simulink model "RaibertControlV9"  (R2022a)
settings: Solver=ode23t  StartTime=0.0  StopTime=10  FixedStep=1/1000  MaxStep=0.001  RelTol=1e-3  AbsTol=1e-3  EnableMultiTasking=on
values from neighbouring files (symbols this model uses):
  dphi_d_14 = 0.0    (= 0)    [initialization.m]
  dphi_d_23 = 0.0    (= 0)    [initialization.m]
  dphi_des = DesiredImpedenceValues(4)    [Controller.m]    (also in initialization.m = 0)
  dr_d_14 = 0.0    (= 0)    [initialization.m]
  dr_d_23 = 0.0    (= 0)    [initialization.m]
  dr_des = DesiredImpedenceValues(3)    [Controller.m]    (also in initialization.m = 0)
  Fpush_d_14 = 300    [initialization.m]
  Fpush_d_23 = 300    [initialization.m]
  GAIN_dx_d_14 = 0.05    [initialization.m]
  GAIN_dx_d_23 = 0.05    [initialization.m]
  Kd_phi_d_14 = 10    [initialization.m]
  Kd_phi_d_23 = 10    [initialization.m]
  Kd_r_d_14 = Kp_r_d_14*0.1    (= 60)    [initialization.m]
  Kd_r_d_23 = Kp_r_d_23*0.1    (= 50)    [initialization.m]
  Kdphi_des = DesiredImpedenceValues(8)    [Controller.m]    (also in initialization.m = 5)
  Kdr_des = DesiredImpedenceValues(6)    [Controller.m]    (also in initialization.m = 700)
  Kp_phi_d_14 = 200    [initialization.m]
  Kp_phi_d_23 = 200    [initialization.m]
  Kp_r_d_14 = 600    [initialization.m]
  Kp_r_d_23 = 500    [initialization.m]
  Kpphi_des = DesiredImpedenceValues(7)    [Controller.m]    (also in initialization.m = 50)
  Kpr_des = DesiredImpedenceValues(5)    [Controller.m]    (also in initialization.m = 700)
  phi_d_14 = 0    [initialization.m]
  phi_d_23 = 0    [initialization.m]
  phi_des = DesiredImpedenceValues(2)    [Controller.m]    (also in initialization.m = 0)
  r_d_14 = 0.38    [initialization.m]
  r_d_23 = 0.38    [initialization.m]
  r_des = DesiredImpedenceValues(1)    [Controller.m]    (also in initialization.m = 0.4)
  rthrust_d_14 = 0.3    [initialization.m]
  rthrust_d_23 = 0.3    [initialization.m]
undefined symbols (not defined in the file or in its folder): Carrier, N, Ring, T, X, Y, Z
libraries: sm_lib x133, nesl_utility x26, Multibody_Parts_Lib x4, fl_lib x4
(part 2 of 8)

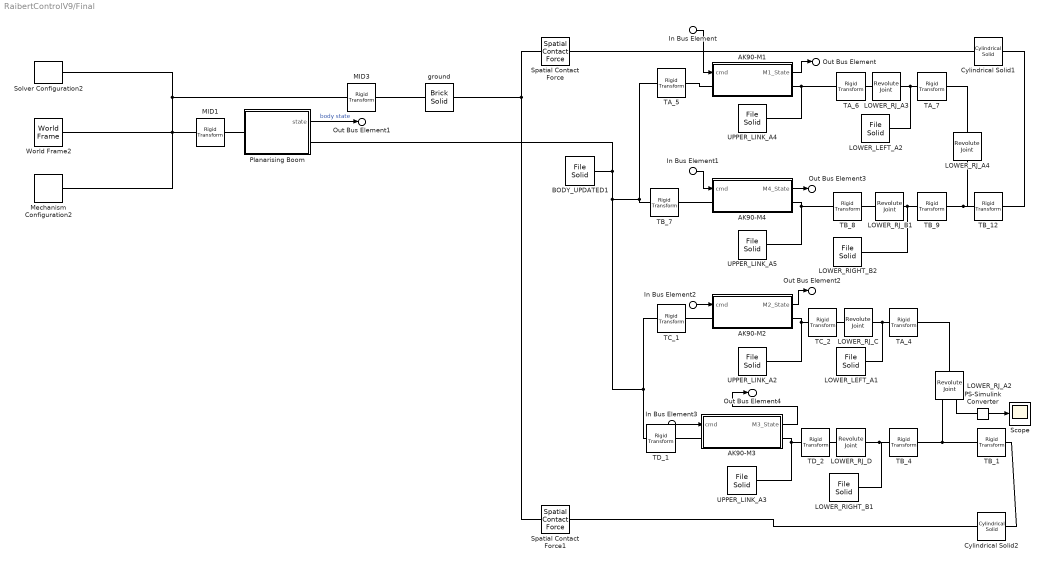
== system RaibertControlV9/Final ==
  In Bus Element1 : Inport  PortName=cmd_M4
  In Bus Element : Inport  Port=2  PortName=cmd_M1
  In Bus Element3 : Inport  Port=3  PortName=cmd_M3
  In Bus Element2 : Inport  Port=4  PortName=cmd_M2
  AK90-M1 : Subsystem
  AK90-M2 : Subsystem
  AK90-M3 : Subsystem
  AK90-M4 : Subsystem
  BODY_UPDATED1 : sm_lib/Body Elements/File Solid  ExtGeomFileName=C:\Users\user\Desktop\Zubair\solidworks_simscape_setup\Rigid Bodies\updated\simscape files\Body.STL  UnitType=Custom  ExtGeomFileUnits=mm  StepReaderType=HEX  ExportConvexHullGeometry=off  InertiaType=Custom  Mass=5756.78  MassUnits=g  CenterOfMass=[0.00 8.34 76.00]  CenterOfMassUnits=mm  MomentsOfInertia="[19417888.32  38930926.54 32124078.52]"  MomentsOfInertiaUnits=g*mm^2  ProductsOfInertia=[0.00 522.32 0.00]  ProductsOfInertiaUnits=g*mm^2  BasedOnType=DensityFromFile  Density=1000  DensityUnits=kg/m^3  DoExposeReferenceFrame=on  SerializedFrames=<Frames/>  GraphicType=FromGeometry  MarkerShape=Sphere  MarkerSize=10  GraphicVisPropType=SimpleVisualProperties  GraphicDiffuseColor=[1.0 1.0 1.0]  GraphicSpecularColor=[0.5 0.5 0.5 1.0]  GraphicAmbientColor=[0.15 0.15 0.15 1.0]  GraphicEmissiveColor=[0.0 0.0 0.0 1.0]  GraphicShininess=75  GraphicOpacity=0.5
  Cylindrical Solid1 : sm_lib/Body Elements/Cylindrical Solid  GraphicAmbientColor=[0.15 0.15 0.15 1.0]  BasedOnType=Density  CenterOfMass=[0 0 0]  CenterOfMassUnits=m  GraphicDiffuseColor=[0.5 0.5 0.5]  CylinderLength=16.25*2  CylinderLengthUnits=mm  CylinderRadius=16.25  CylinderRadiusUnits=mm  Density=1000  DensityUnits=kg/m^3  DoExposeReferenceFrame=on  GraphicEmissiveColor=[0.0 0.0 0.0 1.0]  ExportEntireGeometry=on  SerializedFrames=<Frames/>  MarkerShape=Sphere  MarkerSize=10  GraphicType=FromGeometry  InertiaType=Custom  Mass=0  MassUnits=kg  MomentsOfInertia=[1 1 1]  MomentsOfInertiaUnits=kg*m^2  GraphicOpacity=1.0  ProductsOfInertia=[0 0 0]  ProductsOfInertiaUnits=kg*m^2  GraphicShininess=75  GraphicSpecularColor=[0.5 0.5 0.5 1.0]  GraphicVisPropType=SimpleVisualProperties
  Cylindrical Solid2 : sm_lib/Body Elements/Cylindrical Solid  GraphicAmbientColor=[0.15 0.15 0.15 1.0]  BasedOnType=Density  CenterOfMass=[0 0 0]  CenterOfMassUnits=m  GraphicDiffuseColor=[0.5 0.5 0.5]  CylinderLength=16.25*2  CylinderLengthUnits=mm  CylinderRadius=16.25  CylinderRadiusUnits=mm  Density=1000  DensityUnits=kg/m^3  DoExposeReferenceFrame=on  GraphicEmissiveColor=[0.0 0.0 0.0 1.0]  ExportEntireGeometry=on  SerializedFrames=<Frames/>  MarkerShape=Sphere  MarkerSize=10  GraphicType=FromGeometry  InertiaType=Custom  Mass=0  MassUnits=kg  MomentsOfInertia=[1 1 1]  MomentsOfInertiaUnits=kg*m^2  GraphicOpacity=1.0  ProductsOfInertia=[0 0 0]  ProductsOfInertiaUnits=kg*m^2  GraphicShininess=75  GraphicSpecularColor=[0.5 0.5 0.5 1.0]  GraphicVisPropType=SimpleVisualProperties
  LOWER_LEFT_A1 : sm_lib/Body Elements/File Solid  ExtGeomFileName=C:\Users\user\Desktop\Zubair\solidworks_simscape_setup\Rigid Bodies\updated\simscape files\leg2.STL  UnitType=Custom  ExtGeomFileUnits=mm  StepReaderType=HEX  ExportConvexHullGeometry=off  InertiaType=Custom  Mass=346.45  MassUnits=g  CenterOfMass=[0.00 -132.20 0.00]  CenterOfMassUnits=mm  MomentsOfInertia=[4857689.47 249818.51 4659658.63]  MomentsOfInertiaUnits=g*mm^2  ProductsOfInertia=[0.00 -0.09 10.78]  ProductsOfInertiaUnits=g*mm^2  BasedOnType=DensityFromFile  Density=1000  DensityUnits=kg/m^3  DoExposeReferenceFrame=on  SerializedFrames=<Frames/>  GraphicType=FromGeometry  MarkerShape=Sphere  MarkerSize=10  GraphicVisPropType=SimpleVisualProperties  GraphicDiffuseColor=[1.0 1.0 1.0]  GraphicSpecularColor=[0.5 0.5 0.5 1.0]  GraphicAmbientColor=[0.15 0.15 0.15 1.0]  GraphicEmissiveColor=[0.0 0.0 0.0 1.0]  GraphicShininess=75  GraphicOpacity=1.0
  LOWER_LEFT_A2 : sm_lib/Body Elements/File Solid  ExtGeomFileName=C:\Users\user\Desktop\Zubair\solidworks_simscape_setup\Rigid Bodies\updated\simscape files\leg2.STL  UnitType=Custom  ExtGeomFileUnits=mm  StepReaderType=HEX  ExportConvexHullGeometry=off  InertiaType=Custom  Mass=346.45  MassUnits=g  CenterOfMass=[0.00 -132.20 0.00]  CenterOfMassUnits=mm  MomentsOfInertia=[4857689.47 249818.51 4659658.63]  MomentsOfInertiaUnits=g*mm^2  ProductsOfInertia=[0.00 -0.09 10.78]  ProductsOfInertiaUnits=g*mm^2  BasedOnType=DensityFromFile  Density=1000  DensityUnits=kg/m^3  DoExposeReferenceFrame=on  SerializedFrames=<Frames/>  GraphicType=FromGeometry  MarkerShape=Sphere  MarkerSize=10  GraphicVisPropType=SimpleVisualProperties  GraphicDiffuseColor=[1.0 1.0 1.0]  GraphicSpecularColor=[0.5 0.5 0.5 1.0]  GraphicAmbientColor=[0.15 0.15 0.15 1.0]  GraphicEmissiveColor=[0.0 0.0 0.0 1.0]  GraphicShininess=75  GraphicOpacity=1.0
  LOWER_RIGHT_B1 : sm_lib/Body Elements/File Solid  ExtGeomFileName=C:\Users\user\Desktop\Zubair\solidworks_simscape_setup\Rigid Bodies\updated\simscape files\leg3.STL  UnitType=Custom  ExtGeomFileUnits=mm  StepReaderType=HEX  ExportConvexHullGeometry=off  InertiaType=Custom  Mass=499.95  MassUnits=g  CenterOfMass=[1.63 -190.40 0.00]  CenterOfMassUnits=mm  MomentsOfInertia=[7423471.12 197304.86 7369968.50]  MomentsOfInertiaUnits=g*mm^2  ProductsOfInertia=[2.77 -22.94 255458.86]  ProductsOfInertiaUnits=g*mm^2  BasedOnType=Mass  Density=1000  DensityUnits=kg/m^3  DoExposeReferenceFrame=on  SerializedFrames=<Frames/>  GraphicType=FromGeometry  MarkerShape=Sphere  MarkerSize=10  GraphicVisPropType=SimpleVisualProperties  GraphicDiffuseColor=[1.0 1.0 1.0]  GraphicSpecularColor=[0.5 0.5 0.5 1.0]  GraphicAmbientColor=[0.15 0.15 0.15 1.0]  GraphicEmissiveColor=[0.0 0.0 0.0 1.0]  GraphicShininess=75  GraphicOpacity=1.0
  LOWER_RIGHT_B2 : sm_lib/Body Elements/File Solid  ExtGeomFileName=C:\Users\user\Desktop\Zubair\solidworks_simscape_setup\Rigid Bodies\updated\simscape files\leg3.STL  UnitType=Custom  ExtGeomFileUnits=mm  StepReaderType=HEX  ExportConvexHullGeometry=off  InertiaType=Custom  Mass=499.95  MassUnits=g  CenterOfMass=[1.63 -190.40 0.00]  CenterOfMassUnits=mm  MomentsOfInertia=[7423471.12 197304.86 7369968.50]  MomentsOfInertiaUnits=g*mm^2  ProductsOfInertia=[2.77 -22.94 255458.86]  ProductsOfInertiaUnits=g*mm^2  BasedOnType=Mass  Density=1000  DensityUnits=kg/m^3  DoExposeReferenceFrame=on  SerializedFrames=<Frames/>  GraphicType=FromGeometry  MarkerShape=Sphere  MarkerSize=10  GraphicVisPropType=SimpleVisualProperties  GraphicDiffuseColor=[1.0 1.0 1.0]  GraphicSpecularColor=[0.5 0.5 0.5 1.0]  GraphicAmbientColor=[0.15 0.15 0.15 1.0]  GraphicEmissiveColor=[0.0 0.0 0.0 1.0]  GraphicShininess=75  GraphicOpacity=1.0
  LOWER_RJ_A2 : sm_lib/Joints/Revolute Joint  JointMode=Normal  SenseConstraintForce=off  SenseConstraintForceX=off  SenseConstraintForceY=off  SenseConstraintForceZ=off  SenseConstraintTorque=off  SenseConstraintTorqueX=off  SenseConstraintTorqueY=off  SenseConstraintTorqueZ=off  SenseTotalForce=off  SenseTotalForceX=off  SenseTotalForceY=off  SenseTotalForceZ=off  SenseTotalTorque=off  SenseTotalTorqueX=off  SenseTotalTorqueY=off  SenseTotalTorqueZ=off  CompositeWrenchDir=FollowerOnBase  CompositeWrenchFrame=BaseFrame  EquilibriumPosition=0  EquilibriumPositionUnits=deg  SpringStiffness=0  SpringStiffnessUnits=N*m/deg  DampingCoefficient=0  DampingCoefficientUnits=N*m/(deg/s)  TorqueActuationMode=NoTorque  MotionActuationMode=ComputedMotion  SensePosition=on  SenseVelocity=off  SenseAcceleration=off  SenseTorqueForce=off  SenseLowerLimitTorqueForce=off  SenseUpperLimitTorqueForce=off  LowerLimitSpecify=on  LowerLimitBound=0  LowerLimitBoundUnits=deg  LowerLimitStiffness=1e4  LowerLimitStiffnessUnits=N*m/deg  LowerLimitDamping=10  LowerLimitDampingUnits=N*m/(deg/s)  LowerLimitTransitionRegionWidth=0.1  LowerLimitTransitionRegionWidthUnits=deg  UpperLimitSpecify=off  UpperLimitBound=90  UpperLimitBoundUnits=deg  UpperLimitStiffness=1e4  UpperLimitStiffnessUnits=N*m/deg  UpperLimitDamping=10  UpperLimitDampingUnits=N*m/(deg/s)  UpperLimitTransitionRegionWidth=0.1  UpperLimitTransitionRegionWidthUnits=deg  PositionTargetSpecify=off  PositionTargetPriority=High  PositionTargetValue=10  PositionTargetValueUnits=deg  VelocityTargetSpecify=off  VelocityTargetPriority=High  VelocityTargetValue=0  VelocityTargetValueUnits=deg/s
  LOWER_RJ_A3 : sm_lib/Joints/Revolute Joint  JointMode=Normal  SenseConstraintForce=off  SenseConstraintForceX=off  SenseConstraintForceY=off  SenseConstraintForceZ=off  SenseConstraintTorque=off  SenseConstraintTorqueX=off  SenseConstraintTorqueY=off  SenseConstraintTorqueZ=off  SenseTotalForce=off  SenseTotalForceX=off  SenseTotalForceY=off  SenseTotalForceZ=off  SenseTotalTorque=off  SenseTotalTorqueX=off  SenseTotalTorqueY=off  SenseTotalTorqueZ=off  CompositeWrenchDir=FollowerOnBase  CompositeWrenchFrame=BaseFrame  EquilibriumPosition=0  EquilibriumPositionUnits=deg  SpringStiffness=0  SpringStiffnessUnits=N*m/deg  DampingCoefficient=0  DampingCoefficientUnits=N*m/(deg/s)  TorqueActuationMode=NoTorque  MotionActuationMode=ComputedMotion  SensePosition=off  SenseVelocity=off  SenseAcceleration=off  SenseTorqueForce=off  SenseLowerLimitTorqueForce=off  SenseUpperLimitTorqueForce=off  LowerLimitSpecify=off  LowerLimitBound=-90  LowerLimitBoundUnits=deg  LowerLimitStiffness=1e4  LowerLimitStiffnessUnits=N*m/deg  LowerLimitDamping=10  LowerLimitDampingUnits=N*m/(deg/s)  LowerLimitTransitionRegionWidth=0.1  LowerLimitTransitionRegionWidthUnits=deg  UpperLimitSpecify=off  UpperLimitBound=90  UpperLimitBoundUnits=deg  UpperLimitStiffness=1e4  UpperLimitStiffnessUnits=N*m/deg  UpperLimitDamping=10  UpperLimitDampingUnits=N*m/(deg/s)  UpperLimitTransitionRegionWidth=0.1  UpperLimitTransitionRegionWidthUnits=deg  PositionTargetSpecify=off  PositionTargetPriority=High  PositionTargetValue=10  PositionTargetValueUnits=deg  VelocityTargetSpecify=off  VelocityTargetPriority=High  VelocityTargetValue=0  VelocityTargetValueUnits=deg/s
  LOWER_RJ_A4 : sm_lib/Joints/Revolute Joint  JointMode=Normal  SenseConstraintForce=off  SenseConstraintForceX=off  SenseConstraintForceY=off  SenseConstraintForceZ=off  SenseConstraintTorque=off  SenseConstraintTorqueX=off  SenseConstraintTorqueY=off  SenseConstraintTorqueZ=off  SenseTotalForce=off  SenseTotalForceX=off  SenseTotalForceY=off  SenseTotalForceZ=off  SenseTotalTorque=off  SenseTotalTorqueX=off  SenseTotalTorqueY=off  SenseTotalTorqueZ=off  CompositeWrenchDir=FollowerOnBase  CompositeWrenchFrame=BaseFrame  EquilibriumPosition=0  EquilibriumPositionUnits=deg  SpringStiffness=0  SpringStiffnessUnits=N*m/deg  DampingCoefficient=0  DampingCoefficientUnits=N*m/(deg/s)  TorqueActuationMode=NoTorque  MotionActuationMode=ComputedMotion  SensePosition=off  SenseVelocity=off  SenseAcceleration=off  SenseTorqueForce=off  SenseLowerLimitTorqueForce=off  SenseUpperLimitTorqueForce=off  LowerLimitSpecify=off  LowerLimitBound=0  LowerLimitBoundUnits=deg  LowerLimitStiffness=1e4  LowerLimitStiffnessUnits=N*m/deg  LowerLimitDamping=10  LowerLimitDampingUnits=N*m/(deg/s)  LowerLimitTransitionRegionWidth=0.1  LowerLimitTransitionRegionWidthUnits=deg  UpperLimitSpecify=on  UpperLimitBound=0  UpperLimitBoundUnits=deg  UpperLimitStiffness=1e4  UpperLimitStiffnessUnits=N*m/deg  UpperLimitDamping=10  UpperLimitDampingUnits=N*m/(deg/s)  UpperLimitTransitionRegionWidth=0.1  UpperLimitTransitionRegionWidthUnits=deg  PositionTargetSpecify=off  PositionTargetPriority=High  PositionTargetValue=10  PositionTargetValueUnits=deg  VelocityTargetSpecify=off  VelocityTargetPriority=High  VelocityTargetValue=0  VelocityTargetValueUnits=deg/s
  LOWER_RJ_B1 : sm_lib/Joints/Revolute Joint  JointMode=Normal  SenseConstraintForce=off  SenseConstraintForceX=off  SenseConstraintForceY=off  SenseConstraintForceZ=off  SenseConstraintTorque=off  SenseConstraintTorqueX=off  SenseConstraintTorqueY=off  SenseConstraintTorqueZ=off  SenseTotalForce=off  SenseTotalForceX=off  SenseTotalForceY=off  SenseTotalForceZ=off  SenseTotalTorque=off  SenseTotalTorqueX=off  SenseTotalTorqueY=off  SenseTotalTorqueZ=off  CompositeWrenchDir=FollowerOnBase  CompositeWrenchFrame=BaseFrame  EquilibriumPosition=0  EquilibriumPositionUnits=deg  SpringStiffness=0  SpringStiffnessUnits=N*m/deg  DampingCoefficient=0  DampingCoefficientUnits=N*m/(deg/s)  TorqueActuationMode=NoTorque  MotionActuationMode=ComputedMotion  SensePosition=off  SenseVelocity=off  SenseAcceleration=off  SenseTorqueForce=off  SenseLowerLimitTorqueForce=off  SenseUpperLimitTorqueForce=off  LowerLimitSpecify=off  LowerLimitBound=-90  LowerLimitBoundUnits=deg  LowerLimitStiffness=1e4  LowerLimitStiffnessUnits=N*m/deg  LowerLimitDamping=10  LowerLimitDampingUnits=N*m/(deg/s)  LowerLimitTransitionRegionWidth=0.1  LowerLimitTransitionRegionWidthUnits=deg  UpperLimitSpecify=off  UpperLimitBound=90  UpperLimitBoundUnits=deg  UpperLimitStiffness=1e4  UpperLimitStiffnessUnits=N*m/deg  UpperLimitDamping=10  UpperLimitDampingUnits=N*m/(deg/s)  UpperLimitTransitionRegionWidth=0.1  UpperLimitTransitionRegionWidthUnits=deg  PositionTargetSpecify=off  PositionTargetPriority=High  PositionTargetValue=0  PositionTargetValueUnits=deg  VelocityTargetSpecify=off  VelocityTargetPriority=High  VelocityTargetValue=0  VelocityTargetValueUnits=deg/s
  LOWER_RJ_C : sm_lib/Joints/Revolute Joint  JointMode=Normal  SenseConstraintForce=off  SenseConstraintForceX=off  SenseConstraintForceY=off  SenseConstraintForceZ=off  SenseConstraintTorque=off  SenseConstraintTorqueX=off  SenseConstraintTorqueY=off  SenseConstraintTorqueZ=off  SenseTotalForce=off  SenseTotalForceX=off  SenseTotalForceY=off  SenseTotalForceZ=off  SenseTotalTorque=off  SenseTotalTorqueX=off  SenseTotalTorqueY=off  SenseTotalTorqueZ=off  CompositeWrenchDir=FollowerOnBase  CompositeWrenchFrame=BaseFrame  EquilibriumPosition=0  EquilibriumPositionUnits=deg  SpringStiffness=0  SpringStiffnessUnits=N*m/deg  DampingCoefficient=0  DampingCoefficientUnits=N*m/(deg/s)  TorqueActuationMode=NoTorque  MotionActuationMode=ComputedMotion  SensePosition=off  SenseVelocity=off  SenseAcceleration=off  SenseTorqueForce=off  SenseLowerLimitTorqueForce=off  SenseUpperLimitTorqueForce=off  LowerLimitSpecify=off  LowerLimitBound=-90  LowerLimitBoundUnits=deg  LowerLimitStiffness=1e4  LowerLimitStiffnessUnits=N*m/deg  LowerLimitDamping=10  LowerLimitDampingUnits=N*m/(deg/s)  LowerLimitTransitionRegionWidth=0.1  LowerLimitTransitionRegionWidthUnits=deg  UpperLimitSpecify=off  UpperLimitBound=90  UpperLimitBoundUnits=deg  UpperLimitStiffness=1e4  UpperLimitStiffnessUnits=N*m/deg  UpperLimitDamping=10  UpperLimitDampingUnits=N*m/(deg/s)  UpperLimitTransitionRegionWidth=0.1  UpperLimitTransitionRegionWidthUnits=deg  PositionTargetSpecify=off  PositionTargetPriority=High  PositionTargetValue=10  PositionTargetValueUnits=deg  VelocityTargetSpecify=off  VelocityTargetPriority=High  VelocityTargetValue=0  VelocityTargetValueUnits=deg/s
  LOWER_RJ_D : sm_lib/Joints/Revolute Joint  JointMode=Normal  SenseConstraintForce=off  SenseConstraintForceX=off  SenseConstraintForceY=off  SenseConstraintForceZ=off  SenseConstraintTorque=off  SenseConstraintTorqueX=off  SenseConstraintTorqueY=off  SenseConstraintTorqueZ=off  SenseTotalForce=off  SenseTotalForceX=off  SenseTotalForceY=off  SenseTotalForceZ=off  SenseTotalTorque=off  SenseTotalTorqueX=off  SenseTotalTorqueY=off  SenseTotalTorqueZ=off  CompositeWrenchDir=FollowerOnBase  CompositeWrenchFrame=BaseFrame  EquilibriumPosition=0  EquilibriumPositionUnits=deg  SpringStiffness=0  SpringStiffnessUnits=N*m/deg  DampingCoefficient=0  DampingCoefficientUnits=N*m/(deg/s)  TorqueActuationMode=NoTorque  MotionActuationMode=ComputedMotion  SensePosition=off  SenseVelocity=off  SenseAcceleration=off  SenseTorqueForce=off  SenseLowerLimitTorqueForce=off  SenseUpperLimitTorqueForce=off  LowerLimitSpecify=off  LowerLimitBound=-90  LowerLimitBoundUnits=deg  LowerLimitStiffness=1e4  LowerLimitStiffnessUnits=N*m/deg  LowerLimitDamping=10  LowerLimitDampingUnits=N*m/(deg/s)  LowerLimitTransitionRegionWidth=0.1  LowerLimitTransitionRegionWidthUnits=deg  UpperLimitSpecify=off  UpperLimitBound=90  UpperLimitBoundUnits=deg  UpperLimitStiffness=1e4  UpperLimitStiffnessUnits=N*m/deg  UpperLimitDamping=10  UpperLimitDampingUnits=N*m/(deg/s)  UpperLimitTransitionRegionWidth=0.1  UpperLimitTransitionRegionWidthUnits=deg  PositionTargetSpecify=off  PositionTargetPriority=High  PositionTargetValue=0  PositionTargetValueUnits=deg  VelocityTargetSpecify=off  VelocityTargetPriority=High  VelocityTargetValue=0  VelocityTargetValueUnits=deg/s
  MID1 : sm_lib/Frames and Transforms/Rigid Transform  TranslationMethod=None  TranslationStandardOffset=700  TranslationLengthUnit=mm  TranslationStandardAxis=-Y  TranslationCartesianOffset=[0 0 0]  TranslationROffset=0  TranslationROffsetUnits=m  TranslationZOffset=0  TranslationZOffsetUnits=m  TranslationThetaOffset=0  TranslationThetaOffsetUnits=deg  RotationMethod=StandardAxis  RotationAngleUnits=deg  RotationStandardAxis=+X  RotationAngle=90  RotationArbitraryAxis=[0 0 1]  FollAlignAxisA=+X  BaseAlignAxisA=+Y  FollAlignAxisB=+Y  BaseAlignAxisB=+Z  RotationSequenceAxes=FollowerAxes  RotationSequence=XYX  RotationSequenceAngles=[0 0 0]  RotationSequenceAnglesUnits=deg  RotationMatrix=[1 0 0; 0 1 0; 0 0 1]
  MID3 : sm_lib/Frames and Transforms/Rigid Transform  TranslationMethod=StandardAxis  TranslationStandardOffset=1  TranslationLengthUnit=m  TranslationStandardAxis=-X  TranslationCartesianOffset=[0 0 0]  TranslationROffset=0  TranslationROffsetUnits=m  TranslationZOffset=0  TranslationZOffsetUnits=m  TranslationThetaOffset=0  TranslationThetaOffsetUnits=deg  RotationMethod=StandardAxis  RotationAngleUnits=deg  RotationStandardAxis=+X  RotationAngle=-90  RotationArbitraryAxis=[0 0 1]  FollAlignAxisA=+X  BaseAlignAxisA=+Y  FollAlignAxisB=+Y  BaseAlignAxisB=+Z  RotationSequenceAxes=FollowerAxes  RotationSequence=XYX  RotationSequenceAngles=[0 0 0]  RotationSequenceAnglesUnits=deg  RotationMatrix=[1 0 0; 0 1 0; 0 0 1]
  Mechanism Configuration2 : sm_lib/Utilities/Mechanism Configuration  UniformGravity=Constant  GravityVector=[0 -9.80665 0]  GravityUnits=m/s^2  LinearizationDelta=0.001  JointModeTransitionNonlinearIterations=2
  PS-Simulink Converter : nesl_utility/PS-Simulink Converter  PhysicalDomain=network_engine_domain  SubClassName=ps_output  LeftPortType=input  RightPortType=output  PseudoPeriodic=off  Frequencies=[]  VectorFormat=inherit  Unit=inherit  AffineConversion=off
      settings: SourceProductBaseCode=SS,PW,VE
  Planarising Boom : Subsystem
  Scope : Scope
  Solver Configuration2 : nesl_utility/Solver Configuration  PhysicalDomain=network_engine_domain  SubClassName=solver  LeftPortType=input  RightPortType=generic  Tones=[]  Harmonics=[]  SimulateNoise=off  Profile=off  UseLocalSampling=off  EnableSwitchedLinearOptims=on  FrequencyDomain=off  UseCCode=off  RelTol=0.001  AbsTol=1e-06  MinStep=1e-09  ToWorkspace=off  RevertToSquareIcSolve=off  NumHomotopyIterations=100  PhasorMode=off  PhasorModeNumHarmonics=1  IndexReductionMethod=DerivativeReplacement  DoDC=off  ResidualTolerance=1e-09  UseLocalSolver=off  LocalSolverChoice=NE_BACKWARD_EULER_ADVANCER  LocalSolverSampleTime=0.001  DoFixedCost=off  MaxNonlinIter=3  MaxModeIter=2  ComputeImpulses=off  ImpulseIterations=2  LinearAlgebra=Sparse  LinearAlgebraNumThread=0  EquationFormulation=NE_TIME_EF  DelaysMemoryBudget=1024  AutomaticFiltering=on  FilteringTimeConstant=0.001  PartitionStorageMethod=AS_NEEDED  PartitionMemoryBudget=1024  PartitionMethod=FAST
      settings: SourceProductBaseCode=SS,PW,VE
  Spatial Contact Force : sm_lib/Forces and Torques/Spatial Contact Force  SenseContactBaseRotation=off  SenseContactBaseTranslation=off  CoefficientOfDynamicFriction=0.7  CoefficientOfStaticFriction=0.9  NormalDamping=1e3  NormalDampingUnits=N/(m/s)  SenseContactSignal=off  NormalStiffness=5e4  NormalStiffnessUnits=N/m  FrictionalCriticalVelocity=1e-3  FrictionalCriticalVelocityUnits=m/s  ZeroCrossDetectContactStartAndEnd=on  SenseContactFollowerRotation=off  SenseContactFollowerTranslation=off  FrictionType=SmoothStickSlip  SenseFrictionalForceMagnitude=off  SenseNormalForceMagnitude=off  NormalForceType=SmoothSpringDamper  SenseNormalVelocity=off  SenseSeparationDistance=off  SenseTangentialVelocity=off  NormalTransitionRegionWidth=1e-4  NormalTransitionRegionWidthUnits=m
  Spatial Contact Force1 : sm_lib/Forces and Torques/Spatial Contact Force  SenseContactBaseRotation=off  SenseContactBaseTranslation=off  CoefficientOfDynamicFriction=0.7  CoefficientOfStaticFriction=0.9  NormalDamping=1e3  NormalDampingUnits=N/(m/s)  SenseContactSignal=off  NormalStiffness=5e4  NormalStiffnessUnits=N/m  FrictionalCriticalVelocity=1e-3  FrictionalCriticalVelocityUnits=m/s  ZeroCrossDetectContactStartAndEnd=on  SenseContactFollowerRotation=off  SenseContactFollowerTranslation=off  FrictionType=SmoothStickSlip  SenseFrictionalForceMagnitude=off  SenseNormalForceMagnitude=off  NormalForceType=SmoothSpringDamper  SenseNormalVelocity=off  SenseSeparationDistance=off  SenseTangentialVelocity=off  NormalTransitionRegionWidth=1e-4  NormalTransitionRegionWidthUnits=m
  TA_4 : sm_lib/Frames and Transforms/Rigid Transform  TranslationMethod=Cartesian  TranslationStandardOffset=60  TranslationLengthUnit=mm  TranslationStandardAxis=-X  TranslationCartesianOffset=[0 -300 0]  TranslationROffset=0  TranslationROffsetUnits=m  TranslationZOffset=0  TranslationZOffsetUnits=m  TranslationThetaOffset=0  TranslationThetaOffsetUnits=deg  RotationMethod=None  RotationAngleUnits=deg  RotationStandardAxis=+Z  RotationAngle=0.0  RotationArbitraryAxis=[0 0 1]  FollAlignAxisA=+Y  BaseAlignAxisA=+Y  FollAlignAxisB=+Z  BaseAlignAxisB=+X  RotationSequenceAxes=FollowerAxes  RotationSequence=XYX  RotationSequenceAngles=[0 0 0]  RotationSequenceAnglesUnits=deg  RotationMatrix=[1 0 0; 0 1 0; 0 0 1]
  TA_5 : sm_lib/Frames and Transforms/Rigid Transform  TranslationMethod=StandardAxis  TranslationStandardOffset=60  TranslationLengthUnit=mm  TranslationStandardAxis=+X  TranslationCartesianOffset=[0 0 0]  TranslationROffset=0  TranslationROffsetUnits=m  TranslationZOffset=0  TranslationZOffsetUnits=m  TranslationThetaOffset=0  TranslationThetaOffsetUnits=deg  RotationMethod=AlignedAxes  RotationAngleUnits=deg  RotationStandardAxis=+Z  RotationAngle=0.0  RotationArbitraryAxis=[0 0 1]  FollAlignAxisA=-X  BaseAlignAxisA=+X  FollAlignAxisB=+Z  BaseAlignAxisB=-Z  RotationSequenceAxes=FollowerAxes  RotationSequence=XYX  RotationSequenceAngles=[0 0 0]  RotationSequenceAnglesUnits=deg  RotationMatrix=[1 0 0; 0 1 0; 0 0 1]
  TA_6 : sm_lib/Frames and Transforms/Rigid Transform  TranslationMethod=Cartesian  TranslationStandardOffset=60  TranslationLengthUnit=mm  TranslationStandardAxis=-X  TranslationCartesianOffset=[0 -174.5 34]  TranslationROffset=0  TranslationROffsetUnits=m  TranslationZOffset=0  TranslationZOffsetUnits=m  TranslationThetaOffset=0  TranslationThetaOffsetUnits=deg  RotationMethod=None  RotationAngleUnits=deg  RotationStandardAxis=+Z  RotationAngle=0.0  RotationArbitraryAxis=[0 0 1]  FollAlignAxisA=+Y  BaseAlignAxisA=+Y  FollAlignAxisB=+Z  BaseAlignAxisB=+X  RotationSequenceAxes=FollowerAxes  RotationSequence=XYX  RotationSequenceAngles=[0 0 0]  RotationSequenceAnglesUnits=deg  RotationMatrix=[1 0 0; 0 1 0; 0 0 1]
  TA_7 : sm_lib/Frames and Transforms/Rigid Transform  TranslationMethod=Cartesian  TranslationStandardOffset=60  TranslationLengthUnit=mm  TranslationStandardAxis=-X  TranslationCartesianOffset=[0 -300 0]  TranslationROffset=0  TranslationROffsetUnits=m  TranslationZOffset=0  TranslationZOffsetUnits=m  TranslationThetaOffset=0  TranslationThetaOffsetUnits=deg  RotationMethod=None  RotationAngleUnits=deg  RotationStandardAxis=+Z  RotationAngle=0.0  RotationArbitraryAxis=[0 0 1]  FollAlignAxisA=+Y  BaseAlignAxisA=+Y  FollAlignAxisB=+Z  BaseAlignAxisB=+X  RotationSequenceAxes=FollowerAxes  RotationSequence=XYX  RotationSequenceAngles=[0 0 0]  RotationSequenceAnglesUnits=deg  RotationMatrix=[1 0 0; 0 1 0; 0 0 1]
  TB_1 : sm_lib/Frames and Transforms/Rigid Transform  TranslationMethod=Cartesian  TranslationStandardOffset=60  TranslationLengthUnit=mm  TranslationStandardAxis=-X  TranslationCartesianOffset="[-18.56 -18.56  0]"  TranslationROffset=0  TranslationROffsetUnits=m  TranslationZOffset=0  TranslationZOffsetUnits=m  TranslationThetaOffset=0  TranslationThetaOffsetUnits=deg  RotationMethod=None  RotationAngleUnits=deg  RotationStandardAxis=+Z  RotationAngle=0.0  RotationArbitraryAxis=[0 0 1]  FollAlignAxisA=+Y  BaseAlignAxisA=+Y  FollAlignAxisB=+Z  BaseAlignAxisB=+X  RotationSequenceAxes=FollowerAxes  RotationSequence=XYX  RotationSequenceAngles=[0 0 0]  RotationSequenceAnglesUnits=deg  RotationMatrix=[1 0 0; 0 1 0; 0 0 1]
  TB_12 : sm_lib/Frames and Transforms/Rigid Transform  TranslationMethod=Cartesian  TranslationStandardOffset=60  TranslationLengthUnit=mm  TranslationStandardAxis=-X  TranslationCartesianOffset="[18.56 -18.56  0]"  TranslationROffset=0  TranslationROffsetUnits=m  TranslationZOffset=0  TranslationZOffsetUnits=m  TranslationThetaOffset=0  TranslationThetaOffsetUnits=deg  RotationMethod=None  RotationAngleUnits=deg  RotationStandardAxis=+Z  RotationAngle=0.0  RotationArbitraryAxis=[0 0 1]  FollAlignAxisA=+Y  BaseAlignAxisA=+Y  FollAlignAxisB=+Z  BaseAlignAxisB=+X  RotationSequenceAxes=FollowerAxes  RotationSequence=XYX  RotationSequenceAngles=[0 0 0]  RotationSequenceAnglesUnits=deg  RotationMatrix=[1 0 0; 0 1 0; 0 0 1]
  TB_4 : sm_lib/Frames and Transforms/Rigid Transform  TranslationMethod=Cartesian  TranslationStandardOffset=60  TranslationLengthUnit=mm  TranslationStandardAxis=-X  TranslationCartesianOffset=[0 -295.5 0]  TranslationROffset=0  TranslationROffsetUnits=m  TranslationZOffset=0  TranslationZOffsetUnits=m  TranslationThetaOffset=0  TranslationThetaOffsetUnits=deg  RotationMethod=StandardAxis  RotationAngleUnits=deg  RotationStandardAxis=+Y  RotationAngle=-180.0  RotationArbitraryAxis=[0 0 1]  FollAlignAxisA=+Y  BaseAlignAxisA=+Y  FollAlignAxisB=+Z  BaseAlignAxisB=+X  RotationSequenceAxes=FollowerAxes  RotationSequence=XYX  RotationSequenceAngles=[0 0 0]  RotationSequenceAnglesUnits=deg  RotationMatrix=[1 0 0; 0 1 0; 0 0 1]
  TB_7 : sm_lib/Frames and Transforms/Rigid Transform  TranslationMethod=StandardAxis  TranslationStandardOffset=60  TranslationLengthUnit=mm  TranslationStandardAxis=-X  TranslationCartesianOffset=[0 0 0]  TranslationROffset=0  TranslationROffsetUnits=m  TranslationZOffset=0  TranslationZOffsetUnits=m  TranslationThetaOffset=0  TranslationThetaOffsetUnits=deg  RotationMethod=AlignedAxes  RotationAngleUnits=deg  RotationStandardAxis=+Z  RotationAngle=0.0  RotationArbitraryAxis=[0 0 1]  FollAlignAxisA=-X  BaseAlignAxisA=+X  FollAlignAxisB=+Z  BaseAlignAxisB=-Z  RotationSequenceAxes=FollowerAxes  RotationSequence=XYX  RotationSequenceAngles=[0 0 0]  RotationSequenceAnglesUnits=deg  RotationMatrix=[1 0 0; 0 1 0; 0 0 1]
  TB_8 : sm_lib/Frames and Transforms/Rigid Transform  TranslationMethod=Cartesian  TranslationStandardOffset=60  TranslationLengthUnit=mm  TranslationStandardAxis=-X  TranslationCartesianOffset=[0 -174.5 34]  TranslationROffset=0  TranslationROffsetUnits=m  TranslationZOffset=0  TranslationZOffsetUnits=m  TranslationThetaOffset=0  TranslationThetaOffsetUnits=deg  RotationMethod=None  RotationAngleUnits=deg  RotationStandardAxis=+Z  RotationAngle=0.0  RotationArbitraryAxis=[0 0 1]  FollAlignAxisA=+X  BaseAlignAxisA=-X  FollAlignAxisB=+Y  BaseAlignAxisB=+Y  RotationSequenceAxes=FollowerAxes  RotationSequence=XYX  RotationSequenceAngles=[0 0 0]  RotationSequenceAnglesUnits=deg  RotationMatrix=[1 0 0; 0 1 0; 0 0 1]
  TB_9 : sm_lib/Frames and Transforms/Rigid Transform  TranslationMethod=Cartesian  TranslationStandardOffset=60  TranslationLengthUnit=mm  TranslationStandardAxis=-X  TranslationCartesianOffset=[0 -295.5 0]  TranslationROffset=0  TranslationROffsetUnits=m  TranslationZOffset=0  TranslationZOffsetUnits=m  TranslationThetaOffset=0  TranslationThetaOffsetUnits=deg  RotationMethod=None  RotationAngleUnits=deg  RotationStandardAxis=+Z  RotationAngle=0.0  RotationArbitraryAxis=[0 0 1]  FollAlignAxisA=+Y  BaseAlignAxisA=+Y  FollAlignAxisB=+Z  BaseAlignAxisB=+X  RotationSequenceAxes=FollowerAxes  RotationSequence=XYX  RotationSequenceAngles=[0 0 0]  RotationSequenceAnglesUnits=deg  RotationMatrix=[1 0 0; 0 1 0; 0 0 1]
  TC_1 : sm_lib/Frames and Transforms/Rigid Transform  TranslationMethod=Cartesian  TranslationStandardOffset=60  TranslationLengthUnit=mm  TranslationStandardAxis=+X  TranslationCartesianOffset=[60 0 152]  TranslationROffset=0  TranslationROffsetUnits=m  TranslationZOffset=0  TranslationZOffsetUnits=m  TranslationThetaOffset=0  TranslationThetaOffsetUnits=deg  RotationMethod=None  RotationAngleUnits=deg  RotationStandardAxis=+Z  RotationAngle=0.0  RotationArbitraryAxis=[0 0 1]  FollAlignAxisA=-X  BaseAlignAxisA=+X  FollAlignAxisB=+Z  BaseAlignAxisB=-Z  RotationSequenceAxes=FollowerAxes  RotationSequence=XYX  RotationSequenceAngles=[0 0 0]  RotationSequenceAnglesUnits=deg  RotationMatrix=[1 0 0; 0 1 0; 0 0 1]
  TC_2 : sm_lib/Frames and Transforms/Rigid Transform  TranslationMethod=Cartesian  TranslationStandardOffset=60  TranslationLengthUnit=mm  TranslationStandardAxis=-X  TranslationCartesianOffset=[0 -174.5 34]  TranslationROffset=0  TranslationROffsetUnits=m  TranslationZOffset=0  TranslationZOffsetUnits=m  TranslationThetaOffset=0  TranslationThetaOffsetUnits=deg  RotationMethod=None  RotationAngleUnits=deg  RotationStandardAxis=+Z  RotationAngle=0.0  RotationArbitraryAxis=[0 0 1]  FollAlignAxisA=+Y  BaseAlignAxisA=+Y  FollAlignAxisB=+Z  BaseAlignAxisB=+X  RotationSequenceAxes=FollowerAxes  RotationSequence=XYX  RotationSequenceAngles=[0 0 0]  RotationSequenceAnglesUnits=deg  RotationMatrix=[1 0 0; 0 1 0; 0 0 1]
  TD_1 : sm_lib/Frames and Transforms/Rigid Transform  TranslationMethod=Cartesian  TranslationStandardOffset=60  TranslationLengthUnit=mm  TranslationStandardAxis=-X  TranslationCartesianOffset=[-60 0 152]  TranslationROffset=0  TranslationROffsetUnits=m  TranslationZOffset=0  TranslationZOffsetUnits=m  TranslationThetaOffset=0  TranslationThetaOffsetUnits=deg  RotationMethod=None  RotationAngleUnits=deg  RotationStandardAxis=+Z  RotationAngle=0.0  RotationArbitraryAxis=[0 0 1]  FollAlignAxisA=-X  BaseAlignAxisA=+X  FollAlignAxisB=+Z  BaseAlignAxisB=-Z  RotationSequenceAxes=FollowerAxes  RotationSequence=XYX  RotationSequenceAngles=[0 0 0]  RotationSequenceAnglesUnits=deg  RotationMatrix=[1 0 0; 0 1 0; 0 0 1]
  TD_2 : sm_lib/Frames and Transforms/Rigid Transform  TranslationMethod=Cartesian  TranslationStandardOffset=60  TranslationLengthUnit=mm  TranslationStandardAxis=-X  TranslationCartesianOffset=[0 -174.5 34]  TranslationROffset=0  TranslationROffsetUnits=m  TranslationZOffset=0  TranslationZOffsetUnits=m  TranslationThetaOffset=0  TranslationThetaOffsetUnits=deg  RotationMethod=AlignedAxes  RotationAngleUnits=deg  RotationStandardAxis=+Z  RotationAngle=0.0  RotationArbitraryAxis=[0 0 1]  FollAlignAxisA=+X  BaseAlignAxisA=-X  FollAlignAxisB=+Y  BaseAlignAxisB=+Y  RotationSequenceAxes=FollowerAxes  RotationSequence=XYX  RotationSequenceAngles=[0 0 0]  RotationSequenceAnglesUnits=deg  RotationMatrix=[1 0 0; 0 1 0; 0 0 1]
  UPPER_LINK_A{2..5} (4 alike) : sm_lib/Body Elements/File Solid  ExtGeomFileName=C:\Users\user\Desktop\Zubair\solidworks_simscape_setup\Rigid Bodies\updated\simscape files\leg1.STL  UnitType=Custom  ExtGeomFileUnits=mm  StepReaderType=HEX  ExportConvexHullGeometry=off  InertiaType=Custom  Mass=153.81  MassUnits=g  CenterOfMass=[0.00 -41.14 25.63]  CenterOfMassUnits=mm  MomentsOfInertia=[609040.51 33194.27 600933.68]  MomentsOfInertiaUnits=g*mm^2  ProductsOfInertia=[52980.10 0.00 0.00]  ProductsOfInertiaUnits=g*mm^2  BasedOnType=DensityFromFile  Density=1000  DensityUnits=kg/m^3  DoExposeReferenceFrame=on  SerializedFrames=<Frames/>  GraphicType=FromGeometry  MarkerShape=Sphere  MarkerSize=10  GraphicVisPropType=SimpleVisualProperties  GraphicDiffuseColor=[1.0 1.0 1.0]  GraphicSpecularColor=[0.5 0.5 0.5 1.0]  GraphicAmbientColor=[0.15 0.15 0.15 1.0]  GraphicEmissiveColor=[0.0 0.0 0.0 1.0]  GraphicShininess=75  GraphicOpacity=1.0
  World Frame2 : sm_lib/Frames and Transforms/World Frame
  ground : sm_lib/Body Elements/Brick Solid  GraphicAmbientColor=[0.15 0.15 0.15 1.0]  BasedOnType=Density  BrickDimensions=[4 4 0.0001]  BrickDimensionUnits=m  CenterOfMass=[0 0 0]  CenterOfMassUnits=m  GraphicDiffuseColor=[0.5 0.5 0.5]  Density=1000  DensityUnits=kg/m^3  DoExposeReferenceFrame=on  GraphicEmissiveColor=[0.0 0.0 0.0 1.0]  ExportEntireGeometry=on  SerializedFrames=<Frames/>  MarkerShape=Sphere  MarkerSize=10  GraphicType=FromGeometry  InertiaType=CalculateFromGeometry  Mass=1  MassUnits=kg  MomentsOfInertia=[1 1 1]  MomentsOfInertiaUnits=kg*m^2  GraphicOpacity=1.0  ProductsOfInertia=[0 0 0]  ProductsOfInertiaUnits=kg*m^2  GraphicShininess=75  GraphicSpecularColor=[0.5 0.5 0.5 1.0]  GraphicVisPropType=SimpleVisualProperties
  Out Bus Element3 : Outport  VectorParamsAs1DForOutWhenUnconnected=off  PortName=M4_State
  Out Bus Element : Outport  Port=2  VectorParamsAs1DForOutWhenUnconnected=off  PortName=M1_State
  Out Bus Element4 : Outport  Port=3  VectorParamsAs1DForOutWhenUnconnected=off  PortName=M3_State
  Out Bus Element2 : Outport  Port=4  VectorParamsAs1DForOutWhenUnconnected=off  PortName=M2_State
  Out Bus Element1 : Outport  Port=5  PortName=boom_state
  wires:
  Planarising Boom/1(state) -> Out Bus Element1/1  "body state"
  In Bus Element/1 -> AK90-M1/1(cmd)
  In Bus Element1/1 -> AK90-M4/1(cmd)
  In Bus Element2/1 -> AK90-M2/1(cmd)
  In Bus Element3/1 -> AK90-M3/1(cmd)
  AK90-M1/1(M1_State) -> Out Bus Element/1
  AK90-M4/1(M4_State) -> Out Bus Element3/1
  AK90-M3/1(M3_State) -> Out Bus Element4/1
  AK90-M2/1(M2_State) -> Out Bus Element2/1
  PS-Simulink Converter/1 -> Scope/1
  connections:
  Cylindrical Solid2/RConn1 -- TB_1/RConn1
  LOWER_RJ_A4/RConn1 -- TB_9/RConn1 -- TB_12/LConn1
  TB_9/LConn1 -- LOWER_RIGHT_B2/RConn1 -- LOWER_RJ_B1/RConn1
  TB_4/RConn1 -- TB_1/LConn1 -- LOWER_RJ_A2/RConn1
  Planarising Boom/RConn1 -- TD_1/LConn1 -- TC_1/LConn1 -- TA_5/LConn1 -- TB_7/LConn1 -- BODY_UPDATED1/RConn1
  LOWER_RIGHT_B1/RConn1 -- TB_4/LConn1 -- LOWER_RJ_D/RConn1
  TA_7/LConn1 -- LOWER_LEFT_A2/RConn1 -- LOWER_RJ_A3/RConn1
  UPPER_LINK_A5/RConn1 -- TB_8/LConn1 -- AK90-M4/RConn1
  TA_6/LConn1 -- UPPER_LINK_A4/RConn1 -- AK90-M1/RConn1
  TC_2/RConn1 -- LOWER_RJ_C/LConn1
  AK90-M3/RConn1 -- UPPER_LINK_A3/RConn1 -- TD_2/LConn1
  TD_2/RConn1 -- LOWER_RJ_D/LConn1
  LOWER_LEFT_A1/RConn1 -- TA_4/LConn1 -- LOWER_RJ_C/RConn1
  ground/RConn1 -- MID3/LConn1
  TA_6/RConn1 -- LOWER_RJ_A3/LConn1
  TB_8/RConn1 -- LOWER_RJ_B1/LConn1
  TA_7/RConn1 -- LOWER_RJ_A4/LConn1
  ground/LConn1 -- Spatial Contact Force1/LConn1 -- Spatial Contact Force/LConn1
  Spatial Contact Force/RConn1 -- Cylindrical Solid1/LConn1
  Cylindrical Solid1/RConn1 -- TB_12/RConn1
  AK90-M1/LConn1 -- TA_5/RConn1
  AK90-M4/LConn1 -- TB_7/RConn1
  AK90-M2/LConn1 -- TC_1/RConn1
  Spatial Contact Force1/RConn1 -- Cylindrical Solid2/LConn1
  Planarising Boom/LConn1 -- MID1/LConn1
  LOWER_RJ_A2/LConn1 -- TA_4/RConn1
  AK90-M3/LConn1 -- TD_1/RConn1
  AK90-M2/RConn1 -- UPPER_LINK_A2/RConn1 -- TC_2/LConn1
  Mechanism Configuration2/RConn1 -- MID1/RConn1 -- MID3/RConn1 -- Solver Configuration2/RConn1 -- World Frame2/RConn1
  PS-Simulink Converter/LConn1 -- LOWER_RJ_A2/RConn2

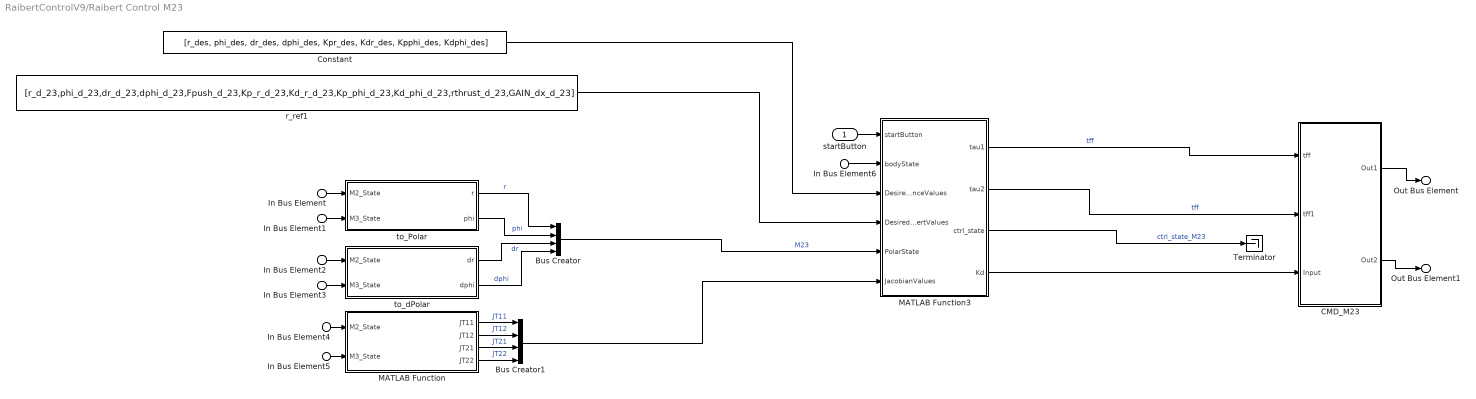
== system RaibertControlV9/Raibert Control M23 ==
  startButton : Inport
  In Bus Element1 : Inport  Port=2  PortName=M3_State
  In Bus Element3 : Inport  Port=2  PortName=M3_State
  In Bus Element5 : Inport  Port=2  PortName=M3_State
  In Bus Element : Inport  Port=3  PortName=M2_State
  In Bus Element2 : Inport  Port=3  PortName=M2_State
  In Bus Element4 : Inport  Port=3  PortName=M2_State
  In Bus Element6 : Inport  Port=4  PortName=bodyState
  Bus Creator : BusCreator  Inputs=4  OutDataTypeStr=Bus: PolarState
      settings: InheritFromInputs=off
  Bus Creator1 : BusCreator  Inputs=4  OutDataTypeStr=Bus: JacobianValues
  CMD_M23 : Subsystem
  Constant : Constant  Value=[r_des, phi_des, dr_des, dphi_des, Kpr_des, Kdr_des, Kpphi_des, Kdphi_des]
  MATLAB Function : MATLAB Function  TreatAsAtomicUnit=on
  MATLAB Function3 : MATLAB Function  TreatAsAtomicUnit=on
  Terminator : Terminator
  r_ref1 : Constant  Value=[r_d_23,phi_d_23,dr_d_23,dphi_d_23,Fpush_d_23,Kp_r_d_23,Kd_r_d_23,Kp_phi_d_23,Kd_phi_d_23,rthrust_d_23,GAIN_dx_d_23]
  to_Polar : MATLAB Function  TreatAsAtomicUnit=on
  to_dPolar : MATLAB Function  TreatAsAtomicUnit=on
  Out Bus Element : Outport  VectorParamsAs1DForOutWhenUnconnected=off  PortName=M3_CMD
  Out Bus Element1 : Outport  Port=2  VectorParamsAs1DForOutWhenUnconnected=off  PortName=M2_CMD
  wires:
  to_Polar/1(r) -> Bus Creator/1  "r"
  to_Polar/2(phi) -> Bus Creator/2  "phi"
  to_dPolar/1(dr) -> Bus Creator/3  "dr"
  to_dPolar/2(dphi) -> Bus Creator/4  "dphi"
  In Bus Element/1 -> to_Polar/1(M2_State)
  In Bus Element1/1 -> to_Polar/2(M3_State)
  In Bus Element2/1 -> to_dPolar/1(M2_State)
  In Bus Element3/1 -> to_dPolar/2(M3_State)
  MATLAB Function/1(JT11) -> Bus Creator1/1  "JT11"
  MATLAB Function/2(JT12) -> Bus Creator1/2  "JT12"
  MATLAB Function/3(JT21) -> Bus Creator1/3  "JT21"
  MATLAB Function/4(JT22) -> Bus Creator1/4  "JT22"
  Bus Creator1/1 -> MATLAB Function3/6(JacobianValues)
  In Bus Element4/1 -> MATLAB Function/1(M2_State)
  In Bus Element5/1 -> MATLAB Function/2(M3_State)
  Bus Creator/1 -> MATLAB Function3/5(PolarState)  "M23"
  In Bus Element6/1 -> MATLAB Function3/2(bodyState)
  MATLAB Function3/1(tau1) -> CMD_M23/1(tff)  "tff"
  MATLAB Function3/2(tau2) -> CMD_M23/2(tff1)  "tff"
  CMD_M23/1(Out1) -> Out Bus Element/1
  CMD_M23/2(Out2) -> Out Bus Element1/1
  startButton/1 -> MATLAB Function3/1(startButton)
  Constant/1 -> MATLAB Function3/3(DesiredImpedenceValues)
  r_ref1/1 -> MATLAB Function3/4(DesiredRaibertValues)
  MATLAB Function3/4(Kd) -> CMD_M23/3(Input)
  MATLAB Function3/3(ctrl_state) -> Terminator/1  "ctrl_state_M23"

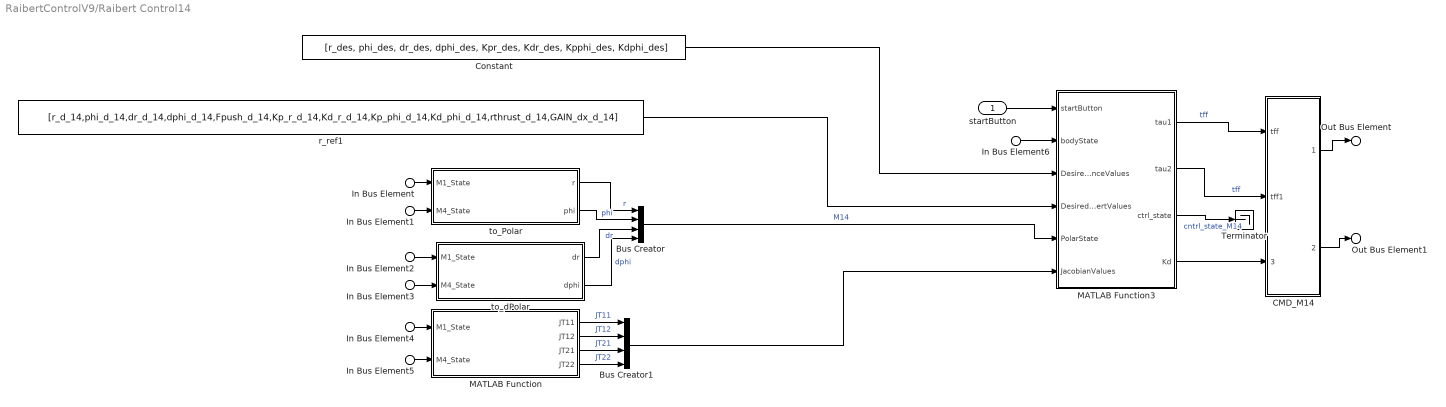
== system RaibertControlV9/Raibert Control14 ==
  startButton : Inport
  In Bus Element1 : Inport  Port=2  PortName=M4_State
  In Bus Element3 : Inport  Port=2  PortName=M4_State
  In Bus Element5 : Inport  Port=2  PortName=M4_State
  In Bus Element : Inport  Port=3  PortName=M1_State
  In Bus Element2 : Inport  Port=3  PortName=M1_State
  In Bus Element4 : Inport  Port=3  PortName=M1_State
  In Bus Element6 : Inport  Port=4  PortName=bodyState
  Bus Creator : BusCreator  Inputs=4  OutDataTypeStr=Bus: PolarState
      settings: InheritFromInputs=off
  Bus Creator1 : BusCreator  Inputs=4  OutDataTypeStr=Bus: JacobianValues
  CMD_M14 : Subsystem
  Constant : Constant  Value=[r_des, phi_des, dr_des, dphi_des, Kpr_des, Kdr_des, Kpphi_des, Kdphi_des]
  MATLAB Function : MATLAB Function  TreatAsAtomicUnit=on
  MATLAB Function3 : MATLAB Function  TreatAsAtomicUnit=on
  Terminator : Terminator
  r_ref1 : Constant  Value=[r_d_14,phi_d_14,dr_d_14,dphi_d_14,Fpush_d_14,Kp_r_d_14,Kd_r_d_14,Kp_phi_d_14,Kd_phi_d_14,rthrust_d_14,GAIN_dx_d_14]
  to_Polar : MATLAB Function  TreatAsAtomicUnit=on
  to_dPolar : MATLAB Function  TreatAsAtomicUnit=on
  Out Bus Element : Outport  VectorParamsAs1DForOutWhenUnconnected=off  PortName=M4_CMD
  Out Bus Element1 : Outport  Port=2  VectorParamsAs1DForOutWhenUnconnected=off  PortName=M1_CMD
  wires:
  to_Polar/1(r) -> Bus Creator/1  "r"
  to_Polar/2(phi) -> Bus Creator/2  "phi"
  to_dPolar/1(dr) -> Bus Creator/3  "dr"
  to_dPolar/2(dphi) -> Bus Creator/4  "dphi"
  In Bus Element/1 -> to_Polar/1(M1_State)
  In Bus Element1/1 -> to_Polar/2(M4_State)
  In Bus Element2/1 -> to_dPolar/1(M1_State)
  In Bus Element3/1 -> to_dPolar/2(M4_State)
  MATLAB Function/1(JT11) -> Bus Creator1/1  "JT11"
  MATLAB Function/2(JT12) -> Bus Creator1/2  "JT12"
  MATLAB Function/3(JT21) -> Bus Creator1/3  "JT21"
  MATLAB Function/4(JT22) -> Bus Creator1/4  "JT22"
  Bus Creator1/1 -> MATLAB Function3/6(JacobianValues)
  In Bus Element4/1 -> MATLAB Function/1(M1_State)
  In Bus Element5/1 -> MATLAB Function/2(M4_State)
  Bus Creator/1 -> MATLAB Function3/5(PolarState)  "M14"
  In Bus Element6/1 -> MATLAB Function3/2(bodyState)
  MATLAB Function3/1(tau1) -> CMD_M14/1(tff)  "tff"
  MATLAB Function3/2(tau2) -> CMD_M14/2(tff1)  "tff"
  CMD_M14/1(Out1) -> Out Bus Element/1
  CMD_M14/2(Out2) -> Out Bus Element1/1
  startButton/1 -> MATLAB Function3/1(startButton)
  MATLAB Function3/3(ctrl_state) -> Terminator/1  "cntrl_state_M14"
  r_ref1/1 -> MATLAB Function3/4(DesiredRaibertValues)
  Constant/1 -> MATLAB Function3/3(DesiredImpedenceValues)
  MATLAB Function3/4(Kd) -> CMD_M14/3(Input)
